simulink model "Model_2"  (R2022b)
settings: Solver=FixedStepAuto  StartTime=0.0  StopTime=inf  RelTol=1e-3
libraries: arduinolib x5
settings Model: ExtModeTrigDuration=2  Creator=djand  LastModifiedBy=djand
settings DataIOCC: ReturnWorkspaceOutputs=off
settings OptimizationCC: EnhancedBackFolding=on  PassReuseOutputArgsAs=Individual arguments  ZeroExternalMemoryAtStartup=off  ZeroInternalMemoryAtStartup=off  MaxStackSize=64  OptimizeBlockOrder=speed  DifferentSizesBufferReuse=on  OptimizationCustomize=off  EfficientTunableParamExpr=on
settings DebuggingCC: ParameterPrecisionLossMsg=none  ParameterTunabilityLossMsg=error
settings HardwareCC: ProdBitPerInt=16  ProdBitPerPointer=16  ProdBitPerSizeT=16  ProdBitPerPtrDiffT=16  ProdLargestAtomicFloat=None  ProdWordSize=8  ProdHWDeviceType=Atmel->AVR
settings SFSimCC: MATLABDynamicMemAlloc=off
settings RTWCC: Description=Embedded Coder  SystemTargetFile=ert.tlc  HardwareBoard=Arduino Uno  TLCOptions=-aInlineSetEventsForThisBaseRateFcn=TLC_FALSE -aSuppressMultiTaskScheduler=TLC_FALSE -aRateBasedStepFcn=1  TemplateMakefile=ert_default_tmf  Toolchain=Arduino AVR  BuildConfiguration=Faster Runs
settings CodeAppCC: ForceParamTrailComments=on  IgnoreCustomStorageClasses=off  OperatorAnnotations=on  SimulinkDataObjDesc=on  SFDataObjDesc=on  InsertBlockDesc=on
settings ERTTargetCC: TargetLangStandard=C99 (ISO)  SupportContinuousTime=on  SupportVariableSizeSignals=on  ExtModeTransport=3  ExtModeStaticAlloc=on  ExtModeAutomaticAllocSize=off  ExtModeStaticAllocSize=250  ExtModeMexFile=ext_xcp  ExtModeIntrfLevel=Level2 - Open

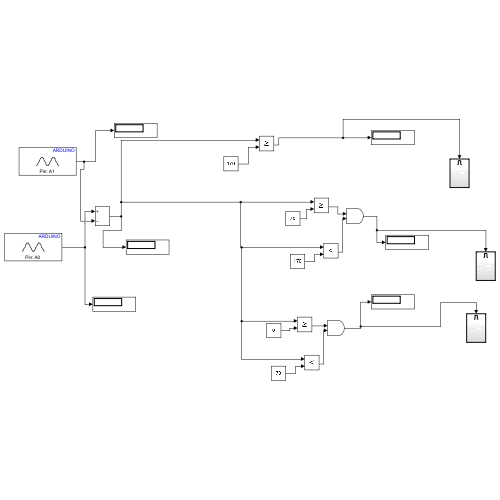
[thumbnail: Simulink's stored preview of the top-level diagram]
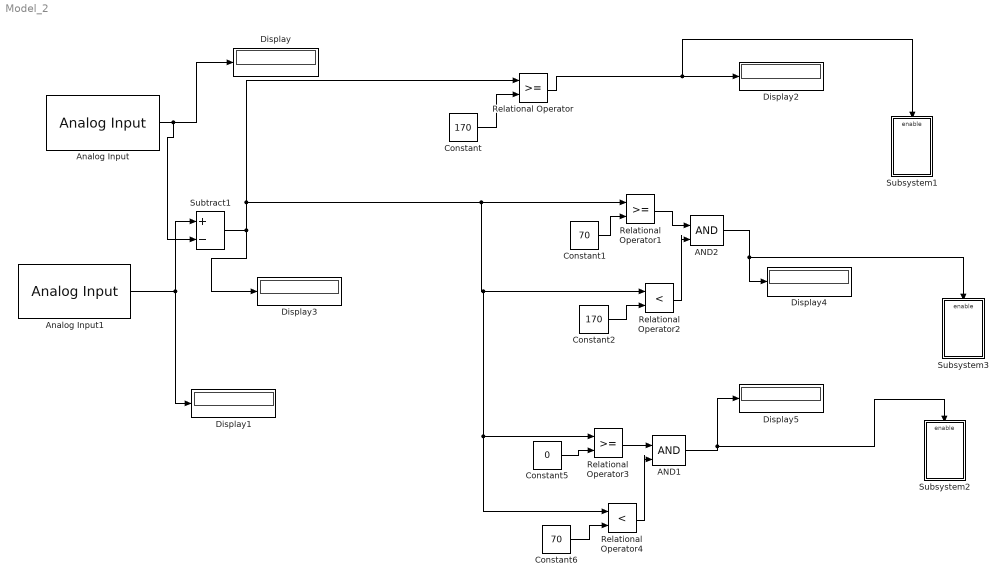
== system Model_2 ==
  AND1 : Logic  IconShape=distinctive  AllPortsSameDT=off  OutDataTypeStr=boolean
  AND2 : Logic  IconShape=distinctive  AllPortsSameDT=off  OutDataTypeStr=boolean
  Analog Input : arduinolib/Analog Input  pinNumber=1  ReadResultsOnly=off  ConversionTriggerSource=Software  ExternalTriggerType=uint32( 0 )  OutputDataType=uint16  EnableConversionCompleteNotify=off  EnableOuputStatus=off  SampleTime=0.1  blockPlatform=arduino
  Analog Input1 : arduinolib/Analog Input  pinNumber=0  ReadResultsOnly=off  ConversionTriggerSource=Software  ExternalTriggerType=uint32( 0 )  OutputDataType=uint16  EnableConversionCompleteNotify=off  EnableOuputStatus=off  SampleTime=0.1  blockPlatform=arduino
  Constant : Constant  Value=170
  Constant1 : Constant  Value=70
  Constant2 : Constant  Value=170
  Constant5 : Constant  Value=0
  Constant6 : Constant  Value=70
  Display{,1..5} (6 alike) : Display
      Display2 settings: Format=decimal (Stored Integer)
      Display3 settings: Format=decimal (Stored Integer)
      Display4 settings: Format=decimal (Stored Integer)
      Display5 settings: Format=decimal (Stored Integer)
  Relational Operator : RelationalOperator  OutDataTypeStr=boolean  RndMeth=Simplest  InputSameDT=off
  Relational Operator1 : RelationalOperator  OutDataTypeStr=boolean  RndMeth=Simplest  InputSameDT=off
  Relational Operator2 : RelationalOperator  Operator=<  OutDataTypeStr=boolean  RndMeth=Simplest  InputSameDT=off
  Relational Operator3 : RelationalOperator  OutDataTypeStr=boolean  RndMeth=Simplest  InputSameDT=off
  Relational Operator4 : RelationalOperator  Operator=<  OutDataTypeStr=boolean  RndMeth=Simplest  InputSameDT=off
  Subsystem1 : Subsystem
  Subsystem2 : Subsystem
  Subsystem3 : Subsystem
  Subtract1 : Sum  Inputs=+-  SaturateOnIntegerOverflow=on  OutDataTypeStr=Inherit: Same as first input
  wires:
  Analog Input/1 -> Display/1, Subtract1/2
  Analog Input1/1 -> Display1/1, Subtract1/1
  Subtract1/1 -> Relational Operator4/1, Relational Operator3/1, Relational Operator2/1, Relational Operator1/1, Relational Operator/1, Display3/1
  Constant/1 -> Relational Operator/2
  Relational Operator2/1 -> AND2/2
  Relational Operator1/1 -> AND2/1
  Constant1/1 -> Relational Operator1/2
  Relational Operator/1 -> Subsystem1/Enable, Display2/1
  AND1/1 -> Subsystem2/Enable, Display5/1
  AND2/1 -> Subsystem3/Enable, Display4/1
  Constant5/1 -> Relational Operator3/2
  Relational Operator3/1 -> AND1/1
  Constant6/1 -> Relational Operator4/2
  Constant2/1 -> Relational Operator2/2
  Relational Operator4/1 -> AND1/2

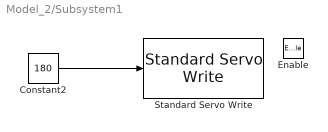
== system Model_2/Subsystem1 ==
  Enable : EnablePort
  Constant2 : Constant  Value=180
  Standard Servo Write : arduinolib/Standard Servo Write  pinNumber=7  ServoIndex=2  blockPlatform=arduino
  wires:
  Constant2/1 -> Standard Servo Write/1

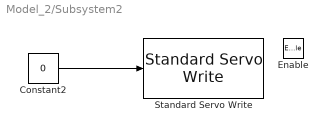
== system Model_2/Subsystem2 ==
  Enable : EnablePort
  Constant2 : Constant  Value=0
  Standard Servo Write : arduinolib/Standard Servo Write  pinNumber=6  ServoIndex=1  blockPlatform=arduino
  wires:
  Constant2/1 -> Standard Servo Write/1

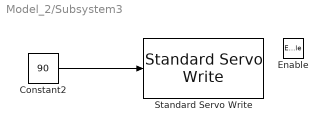
== system Model_2/Subsystem3 ==
  Enable : EnablePort
  Constant2 : Constant  Value=90
  Standard Servo Write : arduinolib/Standard Servo Write  pinNumber=5  ServoIndex=2  blockPlatform=arduino
  wires:
  Constant2/1 -> Standard Servo Write/1
